simulink model "DDC_decimation"  (R2014b)
settings: Solver=FixedStepDiscrete  SolverMode=SingleTasking  StartTime=0.0  StopTime=4096/fs  RelTol=1e-3
PreLoadFcn:
  | %%%%%%%%%%%%%%%%%%%%%%%%%%%%%%%%%%%%%%%%%%%%%%%%%%%%%%%%%%%%%%%%%%%%%%%%%%%
  | % check to see if Simulink library folder is missing from the MATLAB path %
  | %%%%%%%%%%%%%%%%%%%%%%%%%%%%%%%%%%%%%%%%%%%%%%%%%%%%%%%%%%%%%%%%%%%%%%%%%%%
  | if isempty(strfind(path, 'rtlsdr_book_library'))
  | 
  |     % create error window
  |     fig_error = figure(...
  |         'Name', 'Error: RTL-SDR Book Library',...
  |         'Toolbar','none',...
  |         'MenuBar','none',...
  |         'NumberTitle','off',...
  |         'Resize','off',...
  |         'WindowStyle','modal');
  |     fig_error.Position(3) = 600;
  |     fig_error.Position(4) = 150;
  |     fig_axes = axes(...
  |         'Parent',fig_error,...
  |         'Position',[0,0,1,1],...
  |         'visible','off');
  |     % error message
  |     t_title = text(.05,.8,...
  |         'MISSING DIRECTORIES',...
  |         'FontSize',11.5);
  |     t_body = text(.075,.6,...
  |         [{'Simulink cannot find the  \it{<root>}\rm / \it{rtlsdr\_book\_library}\rm  folder in the \it{MATLAB Path}\rm.'},...
  |         {'Please set the MATLAB path following the instructions given in Exercise 2.4.'}],...
  |         'FontSize',10.5);
  |     % buttons
  |     btn_path = uicontrol(...
  |         'Parent',fig_error,...
  |         'String','Set Path Now',...
  |         'FontSize',10,...
  |         'Callback', 'pathtool; close(fig_error);',...
  |         'Position', [fig_error.Position(3)/2-210, 30, 200, 30]);
  |     btn_abort = uicontrol(...
  |         'Parent',fig_error,...
  |         'String','No thanks',...
  |         'FontSize',10,...
  |         'Callback', 'close(fig_error); abort=1;',...
  |         'Position', [fig_error.Position(3)/2+10, 30, 200, 30]);
  | 
  |     % pause to allow user to interact with error box
  |     uiwait(fig_error);
  | 
  |     % abort simulation
  |     try
  |         if abort==1
  |             set_param(gcs, 'SimulationCommand', 'stop');
  |         end
  |     end
  | 
  |     % if user has set path, allow diagram to be updated
  |     if ~exist('abort','var')
  |         % create error window
  |         fig_update = figure(...
  |             'Name', 'Update Diagram',...
  |             'Toolbar','none',...
  |             'MenuBar','none',...
  |             'NumberTitle','off',...
  |             'Resize','off');
  |         fig_update.Position(3) = 400;
  |         fig_update.Position(4) = 120;
  |         fig_axes = axes(...
  |             'Parent',fig_update,...
  |             'Position',[0,0,1,1],...
  |             'visible','off');
  |         % instruction message
  |         t_body = text(.075,.7,...
  |             'Once you have set the path, update the block diagram',...
  |             'FontSize',10.5);
  |         % button
  |         btn_update = uicontrol(...
  |             'Parent',fig_update,...
  |             'String','Update Block Diagram',...
  |             'FontSize',10,...
  |             'Callback', 'set_param(gcs,''SimulationCommand'',''update''); close(gcf)',...
  |             'Position', [fig_update.Position(3)/2-100, 30, 200, 30]);
  |     end
  | 
  |     % clear error components
  |     clear('fig_error','fig_update','fig_axes','t_title','t_body','btn_path','btn_abort','btn_update','abort');
  | 
  | end
  | %%%%%%%%%%%%%%%%%%%%%%%%%%%%%%%%%%%%%%%%%%%%%%%%%%%%%%%%%%%%%%%%%%%%%%%%%%%
  | 
  | DDC1_setup
  | 
  | % annotations for the pink and purple blocks
  | % going from right to left...
  | 
  | MHz = 100;
  | fs = MHz * 1e6;
  | 
  | fs_CIC_in = fs/CIC_R;
  | MHz_CIC_in = MHz/CIC_R;
  | 
  | fs_CFIR_in = fs/(CIC_R*CFIR_L_factor);
  | MHz_CFIR_in = MHz/(CIC_R*CFIR_L_factor);
  | 
  | fs_RRC_in = fs/(CIC_R*CFIR_L_factor*RRC_L_factor);
  | MHz_RRC_in = MHz/(CIC_R*CFIR_L_factor*RRC_L_factor);
StartFcn:
  | close all;
undefined symbols (not defined in the file): CFIR_L_factor, CIC_R, RRC_L_factor, startfcn_time_scope
libraries: dspmlti4 x12, commdigbbndpm3 x2, dspsigops x2, rtlsdr_book_library x1, dsparch4 x1, commnoisgen2 x1, commrandsrc2 x1
CloseFcn:
  | closefcn_model;
Description:
  | Software, Simulation Examples and Design Exercises Licence Agreement
  | 
  | This license agreement refers to the simulation examples, design exercises and files,
  | and associated software MATLAB and Simulink resources that accompany the book:
  | 
  |      Title: Software Defined Radio using MATLAB & Simulink and the RTL-SDR
  |      Published by Strathclyde Academic Media, 2015
  |      Authored by Robert W. Stewart, Kenneth W. Barlee, Dale S.W. Atkinson,
  |      and Louise H. Crockett
  | 
  | and made available as a download from, www.desktopSDR.com or variously acquired
  | by other means such as via USB storage, cloud storage, disk or any other electronic
  | or optical or magnetic storage mechanism. These files and associated software may
  | be used subject to the terms of agreement of the conditions below:
  | 
  |     Copyright © 2015 Robert W. Stewart, Kenneth W. Barlee, Dale S.W. Atkinson,
  |     and Louise H. Crockett
  |     All rights reserved.
  | 
  | Redistribution and use in source and binary forms, with or without modification, are
  | permitted provided that the following conditions are met:
  | 
  |    1.  Redistributions of source code must retain the above copyright notice, this list of
  |         conditions and the following disclaimer.
  | 
  |    2.  Redistributions in binary form must reproduce the above copyright notice, this
  |         list of conditions and the following disclaimer in the documentation and/or other
  |         materials provided with the distribution.
  | 
  |    3.  Neither the name of the copyright holder nor the names of its contributors may
  |         be used to endorse or promote products derived from this software without
  |         specific prior written permission.
  | 
  |    4.  In all cases, the software is, and all modifications and derivatives of the
  |         software shall be, licensed to you solely for use in conjunction with The
  |         MathWorks, Inc. products and service offerings.
  | 
  | THIS SOFTWARE IS PROVIDED BY THE COPYRIGHT HOLDERS AND CONTRIBUTORS
  | "AS IS" AND ANY EXPRESS OR IMPLIED WARRANTIES, INCLUDING, BUT NOT LIMITED
  | TO, THE IMPLIED WARRANTIES OF MERCHANTABILITY AND FITNESS FOR A
  | PARTICULAR PURPOSE ARE DISCLAIMED. IN NO EVENT SHALL THE COPYRIGHT
  | HOLDER OR CONTRIBUTORS BE LIABLE FOR ANY DIRECT, INDIRECT, INCIDENTAL,
  | SPECIAL, EXEMPLARY, OR CONSEQUENTIAL DAMAGES (INCLUDING, BUT NOT
  | LIMITED TO, PROCUREMENT OF SUBSTITUTE GOODS OR SERVICES; LOSS OF USE,
  | DATA, OR PROFITS; OR BUSINESS INTERRUPTION) HOWEVER CAUSED AND ON ANY
  | THEORY OF LIABILITY, WHETHER IN CONTRACT, STRICT LIABILITY, OR TORT
  | (INCLUDING NEGLIGENCE OR OTHERWISE) ARISING IN ANY WAY OUT OF THE USE
  | OF THIS SOFTWARE, EVEN IF ADVISED OF THE POSSIBILITY OF SUCH DAMAGE.
  | 
  | 
  | Audio Tracks used in Simulations Examples and Design Exercises
  | 
  | The music and vocal files used within the Examples files and software within the book
  | were variously written, arranged, performed, recorded and produced by Garrey Rice,
  | Adam Struth, Jamie Struth, Iain Thistlethwaite and also Marshall Craigmyle who
  | collectively, and individually where appropriate, assert and retain all of their copyright,
  | performance and artistic rights. Permission to use and reproduce this music is
  | granted for all purposes associated with MATLAB and Simulink software and the
  | simulation examples and design exercises files that accompany this book. Requests to
  | use the music for any other purpose should be directed to: info@desktopSDR.com.
  | For information on music track names, full credits, and links to the musicians please
  | refer to www.desktopSDR.com/more/audio.
settings Model: Creator=desktopSDR Team  LastModifiedBy=desktopSDR Team
settings DataIOCC: LimitDataPoints=off  SaveOutput=off  SignalLogging=off  SaveTime=off
settings OptimizationCC: BlockReduction=off  ConditionallyExecuteInputs=off  InlineParams=on
settings DebuggingCC: AlgebraicLoopMsg=error  UnderspecifiedInitializationDetection=Classic  MergeDetectMultiDrivingBlocksExec=none  SingleTaskRateTransMsg=error  ParameterOverflowMsg=warning  StateNameClashWarn=warning
settings HardwareCC: ProdHWDeviceType=ASIC/FPGA->ASIC/FPGA  ProdEqTarget=off

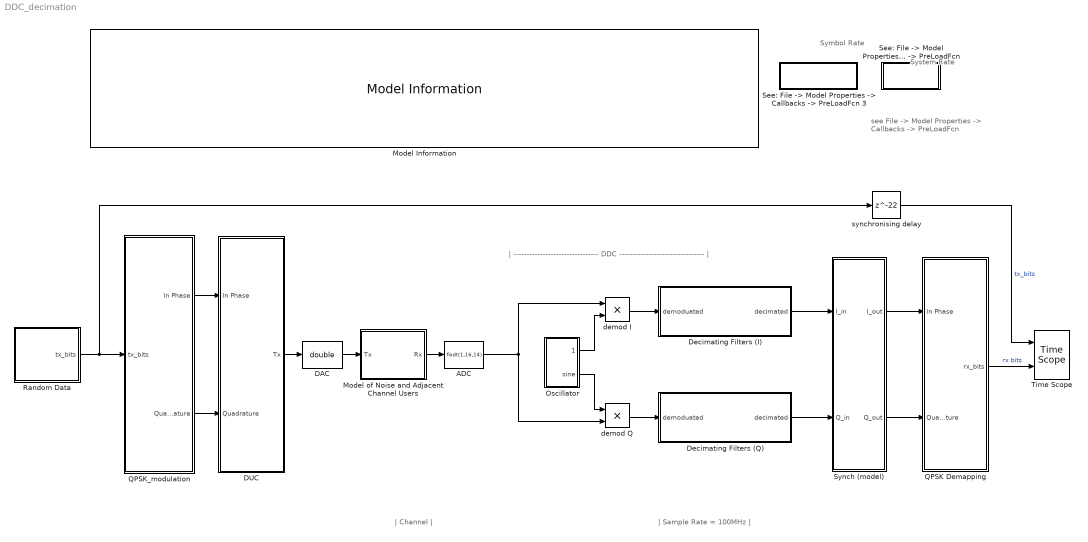
== system DDC_decimation ==
  note: | -------------------------------- DDC -------------------------------- |
  note: System Rate
  note: see File -> Model Properties
      | -> Callbacks -> PreLoadFcn
  note: Symbol Rate
  note: | Sample Rate = 100MHz |
  note: | Channel |
  ADC : DataTypeConversion  OutDataTypeStr=fixdt(1,16,14)
  DAC : DataTypeConversion  OutDataTypeStr=double
  DUC : Subsystem
  Decimating Filters (I) : Subsystem
  Decimating Filters (Q) : Subsystem
  Model Information : rtlsdr_book_library/Additional Tools/Model Information/Model Information
  Model of Noise and Adjacent Channel Users : Subsystem
  Oscillator : Subsystem  mask(Simple Quadrature Oscillator){fc=40e6}
      mask prompts: fc "Frequency"
  QPSK Demapping : Subsystem
  QPSK_modulation : Subsystem
  Random Data : Subsystem
  "See: File -> Model Properties -> Callbacks -> PreLoadFcn " : Subsystem
      mask Display:
      | MHz = evalin('base', 'MHz');
      | fprintf(['fs = ',num2str(MHz),' MHz']);
  "See: File -> Model Properties -> Callbacks -> PreLoadFcn 3" : Subsystem
      mask Display:
      | MHz_RRC_in = evalin('base', 'MHz_RRC_in');
      | fprintf(['fR1 = ',num2str(MHz_RRC_in),' MHz']);
  Synch (model) : Subsystem
  Time Scope : TimeScope  StartFcn=startfcn_time_scope;  DefaultConfigurationName=spbscopes.TimeScopeBlockCfg  NumInputPorts=2
  demod I : Product  OutDataTypeStr=fixdt(1,16,15)
  demod Q : Product  OutDataTypeStr=fixdt(1,16,15)
  synchronising delay : Delay  DelayLength=22  InputProcessing=Columns as channels (frame based)
  wires:
  Random Data/1(tx_bits) -> synchronising delay/1, QPSK_modulation/1(tx_bits)
  ADC/1 -> demod I/1, demod Q/2
  Oscillator/1(cosine) -> demod I/2
  Oscillator/2(sine) -> demod Q/1
  demod I/1 -> Decimating Filters (I)/1(demoduated)
  demod Q/1 -> Decimating Filters (Q)/1(demoduated)
  DAC/1 -> Model of Noise and Adjacent Channel Users/1(Tx)
  QPSK_modulation/1(In Phase) -> DUC/1(In Phase)
  QPSK_modulation/2(Quadrature) -> DUC/2(Quadrature)
  DUC/1(Tx) -> DAC/1
  Model of Noise and Adjacent Channel Users/1(Rx) -> ADC/1
  synchronising delay/1 -> Time Scope/1  "tx_bits"
  QPSK Demapping/1(rx_bits) -> Time Scope/2  "rx bits"
  Decimating Filters (I)/1(" decimated") -> Synch (model)/1(I_in)
  Decimating Filters (Q)/1(" decimated") -> Synch (model)/2(Q_in)
  Synch (model)/1(I_out) -> QPSK Demapping/1(In Phase)
  Synch (model)/2(Q_out) -> QPSK Demapping/2(Quadrature)

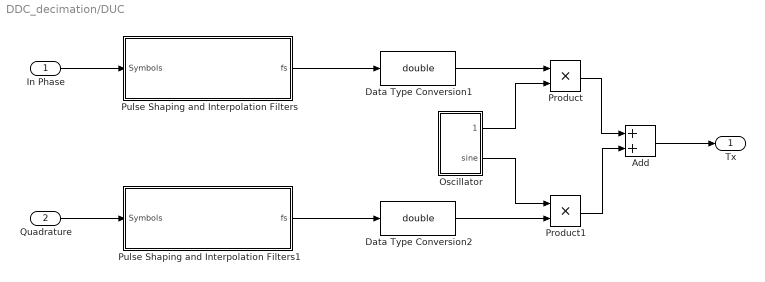
== system DDC_decimation/DUC ==
  In Phase : Inport
  Quadrature : Inport  Port=2
  Add : Sum  OutDataTypeStr=double
  Data Type Conversion1 : DataTypeConversion  OutDataTypeStr=double
  Data Type Conversion2 : DataTypeConversion  OutDataTypeStr=double
  Oscillator : Subsystem  mask(Simple Quadrature Oscillator){fc=40e6}
      mask prompts: fc "Frequency"
  Product : Product  OutDataTypeStr=double
  Product1 : Product  OutDataTypeStr=double
  Pulse Shaping and Interpolation Filters : Subsystem
  Pulse Shaping and Interpolation Filters1 : Subsystem
  Tx : Outport
  wires:
  Add/1 -> Tx/1
  Pulse Shaping and Interpolation Filters/1(" fs") -> Data Type Conversion1/1
  Pulse Shaping and Interpolation Filters1/1(" fs") -> Data Type Conversion2/1
  Oscillator/1(cosine) -> Product/2
  Oscillator/2(sine) -> Product1/1
  Product1/1 -> Add/2
  Product/1 -> Add/1
  Data Type Conversion1/1 -> Product/1
  Data Type Conversion2/1 -> Product1/2
  In Phase/1 -> Pulse Shaping and Interpolation Filters/1(Symbols)
  Quadrature/1 -> Pulse Shaping and Interpolation Filters1/1(Symbols)

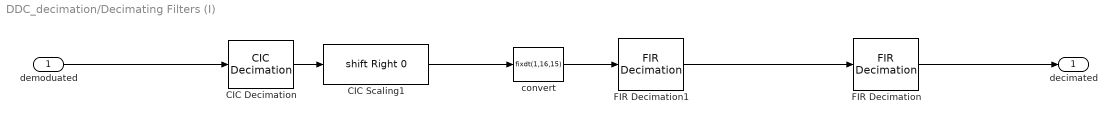
== system DDC_decimation/Decimating Filters (I) ==
  demoduated : Inport
  CIC Decimation : dspmlti4/CIC Decimation  filtFrom=Multirate object in workspace  filtobj=D_hCIC  ftype=Decimator  R=2  M=1  N=2  filterInternals=Full precision  BPS=[16 16 16 16]  FLPS=0  outputWordLength=32  outputFracLength=0  launchFVT=off  framing=Maintain input frame rate  RateOptions=Allow multirate processing
  CIC Scaling1 : ArithShift  BinPtShiftNumber=-10  BitShiftDirection=Right
  FIR Decimation : dspmlti4/FIR Decimation  h=fir1(35,0.4)  D=2  filtStruct=Direct form  framing=Allow multirate processing  inputOffset=0  outputBufInitCond=0  firstCoeffDataTypeStr=Inherit: Same word length as input  firstCoeffLastDataTypeStr=Inherit: Same word length as input  firstCoeffMin=[]  firstCoeffMax=[]  outputDataTypeStr=Inherit: Same as accumulator  outputLastDataTypeStr=Inherit: Same as accumulator  outputMin=[]  outputMax=[]  roundingMode=Floor  overflowMode=off  FilterSource=Filter object  FilterObject=D_hRRC
      settings: allowOverrides=off
  FIR Decimation1 : dspmlti4/FIR Decimation  h=fir1(35,0.4)  D=2  filtStruct=Direct form  framing=Allow multirate processing  inputOffset=0  outputBufInitCond=0  firstCoeffDataTypeStr=Inherit: Same word length as input  firstCoeffLastDataTypeStr=Inherit: Same word length as input  firstCoeffMin=[]  firstCoeffMax=[]  outputDataTypeStr=Inherit: Same as accumulator  outputLastDataTypeStr=Inherit: Same as accumulator  outputMin=[]  outputMax=[]  roundingMode=Floor  overflowMode=off  FilterSource=Filter object  FilterObject=D_hCFIR
      settings: allowOverrides=off
  convert : DataTypeConversion  OutDataTypeStr=fixdt(1,16,15)
  " decimated" : Outport
  wires:
  CIC Decimation/1 -> CIC Scaling1/1
  CIC Scaling1/1 -> convert/1
  FIR Decimation1/1 -> FIR Decimation/1
  demoduated/1 -> CIC Decimation/1
  FIR Decimation/1 -> " decimated"/1
  convert/1 -> FIR Decimation1/1

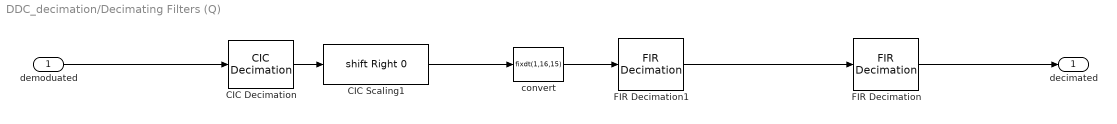
== system DDC_decimation/Decimating Filters (Q) ==
  demoduated : Inport
  CIC Decimation : dspmlti4/CIC Decimation  filtFrom=Multirate object in workspace  filtobj=D_hCIC  ftype=Decimator  R=2  M=1  N=2  filterInternals=Full precision  BPS=[16 16 16 16]  FLPS=0  outputWordLength=32  outputFracLength=0  launchFVT=off  framing=Maintain input frame rate  RateOptions=Allow multirate processing
  CIC Scaling1 : ArithShift  BinPtShiftNumber=-10  BitShiftDirection=Right
  FIR Decimation : dspmlti4/FIR Decimation  h=fir1(35,0.4)  D=2  filtStruct=Direct form  framing=Allow multirate processing  inputOffset=0  outputBufInitCond=0  firstCoeffDataTypeStr=Inherit: Same word length as input  firstCoeffLastDataTypeStr=Inherit: Same word length as input  firstCoeffMin=[]  firstCoeffMax=[]  outputDataTypeStr=Inherit: Same as accumulator  outputLastDataTypeStr=Inherit: Same as accumulator  outputMin=[]  outputMax=[]  roundingMode=Floor  overflowMode=off  FilterSource=Filter object  FilterObject=D_hRRC
      settings: allowOverrides=off
  FIR Decimation1 : dspmlti4/FIR Decimation  h=fir1(35,0.4)  D=2  filtStruct=Direct form  framing=Allow multirate processing  inputOffset=0  outputBufInitCond=0  firstCoeffDataTypeStr=Inherit: Same word length as input  firstCoeffLastDataTypeStr=Inherit: Same word length as input  firstCoeffMin=[]  firstCoeffMax=[]  outputDataTypeStr=Inherit: Same as accumulator  outputLastDataTypeStr=Inherit: Same as accumulator  outputMin=[]  outputMax=[]  roundingMode=Floor  overflowMode=off  FilterSource=Filter object  FilterObject=D_hCFIR
      settings: allowOverrides=off
  convert : DataTypeConversion  OutDataTypeStr=fixdt(1,16,15)
  " decimated" : Outport
  wires:
  FIR Decimation/1 -> " decimated"/1
  demoduated/1 -> CIC Decimation/1
  FIR Decimation1/1 -> FIR Decimation/1
  CIC Scaling1/1 -> convert/1
  CIC Decimation/1 -> CIC Scaling1/1
  convert/1 -> FIR Decimation1/1

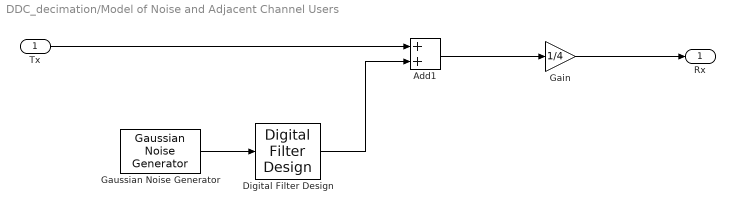
== system DDC_decimation/Model of Noise and Adjacent Channel Users ==
  Tx : Inport
  Add1 : Sum  OutDataTypeStr=fixdt(1,17,14)
  Digital Filter Design : dsparch4/Digital Filter Design  mwdsp_browser_bugfix_var=off
  Gain : Gain  Gain=1/4
  Gaussian Noise Generator : commnoisgen2/Gaussian Noise Generator  m=0  d=1  s=41  Ts=1/fs  frameBased=off  sampPerFrame=1  orient=off  outDataType=double
  Rx : Outport
  wires:
  Tx/1 -> Add1/1
  Gaussian Noise Generator/1 -> Digital Filter Design/1
  Add1/1 -> Gain/1
  Gain/1 -> Rx/1
  Digital Filter Design/1 -> Add1/2

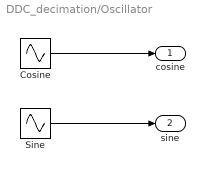
== system DDC_decimation/Oscillator ==
  "Cosine " : Sin  Frequency=fc*2*pi  Phase=pi/2  SampleTime=1/fs
  Sine : Sin  Frequency=fc*2*pi  SampleTime=1/fs
  cosine : Outport
  sine : Outport  Port=2
  wires:
  Sine/1 -> sine/1
  "Cosine "/1 -> cosine/1

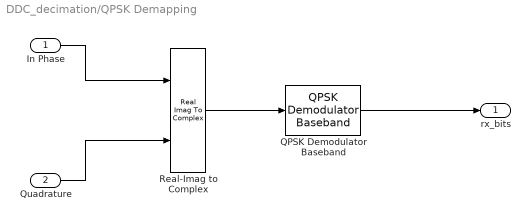
== system DDC_decimation/QPSK Demapping ==
  In Phase : Inport
  Quadrature : Inport  Port=2
  QPSK Demodulator Baseband : commdigbbndpm3/QPSK Demodulator Baseband  Ph=pi/4  Dec=Gray  OutType=Bit  DecType=Hard decision  VarSource=Dialog  Variance=1  outDtype1=Inherit via internal rule  outDtype2=Inherit via internal rule  derotateFactorWordLen=16
  Real-Imag to Complex : RealImagToComplex
  rx_bits : Outport
  wires:
  Quadrature/1 -> Real-Imag to Complex/2
  In Phase/1 -> Real-Imag to Complex/1
  Real-Imag to Complex/1 -> QPSK Demodulator Baseband/1
  QPSK Demodulator Baseband/1 -> rx_bits/1

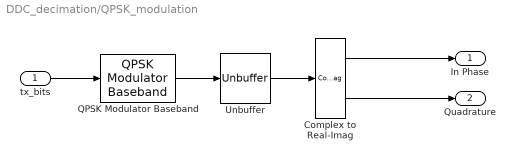
== system DDC_decimation/QPSK_modulation ==
  tx_bits : Inport
  Complex to Real-Imag : ComplexToRealImag
  QPSK Modulator Baseband : commdigbbndpm3/QPSK Modulator Baseband  InType=Bit  Enc=Gray  Ph=pi/4  outDtype=Fixed-point  outWordLen=16  outUDDataType=sfix(16)  outFracLenMode=User-defined  outFracLen=15
  Unbuffer : Unbuffer  SampleBasedProcessing=Same as frame based
  In Phase : Outport
  Quadrature : Outport  Port=2
  wires:
  Complex to Real-Imag/2 -> Quadrature/1
  Complex to Real-Imag/1 -> In Phase/1
  QPSK Modulator Baseband/1 -> Unbuffer/1
  tx_bits/1 -> QPSK Modulator Baseband/1
  Unbuffer/1 -> Complex to Real-Imag/1

== system DDC_decimation/Random Data ==
  Bernoulli Binary Generator : commrandsrc2/Bernoulli Binary Generator  P=0.5  seed=61  Ts=(0.5*CIC_R*RRC_L_factor*CFIR_L_factor)/fs  frameBased=on  sampPerFrame=2  orient=off  outDataType=boolean
  tx_bits : Outport
  wires:
  Bernoulli Binary Generator/1 -> tx_bits/1  "Transmitted Bits"

== system DDC_decimation/See: File -> Model Properties -> Callbacks -> PreLoadFcn  ==

== system DDC_decimation/See: File -> Model Properties -> Callbacks -> PreLoadFcn 3 ==

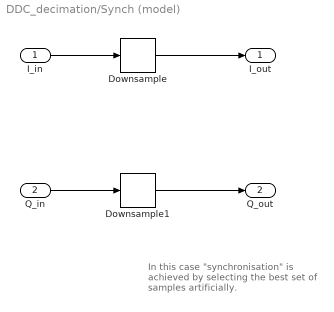
== system DDC_decimation/Synch (model) ==
  note: In this case "synchronisation" is
      | achieved by selecting the best set
      | of samples artificially.
  I_in : Inport
  Q_in : Inport  Port=2
  Downsample : dspsigops/Downsample  N=2  phase=0  RateOptions=Allow multirate processing  smode=Allow multirate  fmode=Maintain input frame size  ic=0
  Downsample1 : dspsigops/Downsample  N=2  phase=0  RateOptions=Allow multirate processing  smode=Allow multirate  fmode=Maintain input frame size  ic=0
  I_out : Outport
  Q_out : Outport  Port=2
  wires:
  I_in/1 -> Downsample/1
  Q_in/1 -> Downsample1/1
  Downsample1/1 -> Q_out/1
  Downsample/1 -> I_out/1

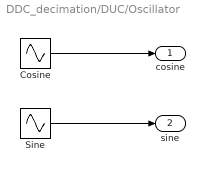
== system DDC_decimation/DUC/Oscillator ==
  "Cosine " : Sin  Frequency=fc*2*pi  Phase=pi/2  SampleTime=1/fs
  Sine : Sin  Frequency=fc*2*pi  SampleTime=1/fs
  cosine : Outport
  sine : Outport  Port=2
  wires:
  Sine/1 -> sine/1
  "Cosine "/1 -> cosine/1

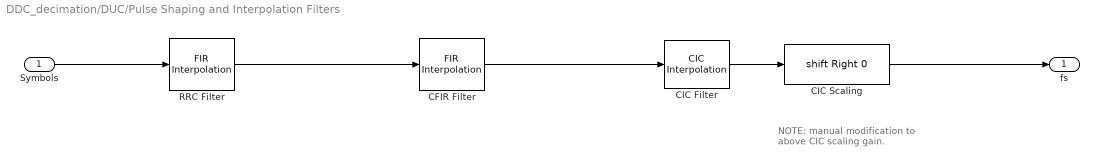
== system DDC_decimation/DUC/Pulse Shaping and Interpolation Filters ==
  note: NOTE: manual modification
      |  to above CIC scaling gain.
  Symbols : Inport
  CFIR Filter : dspmlti4/FIR Interpolation  h=fir1(15,1/4)  L=3  framing=Allow multirate processing  outputBufInitCond=0  firstCoeffDataTypeStr=Inherit: Same word length as input  firstCoeffLastDataTypeStr=Inherit: Same word length as input  firstCoeffMin=[]  firstCoeffMax=[]  outputDataTypeStr=Inherit: Same as accumulator  outputLastDataTypeStr=Inherit: Same as accumulator  outputMin=[]  outputMax=[]  roundingMode=Floor  overflowMode=off  FilterSource=Filter object  FilterObject=hCFIR
  CIC Filter : dspmlti4/CIC Interpolation  filtFrom=Multirate object in workspace  filtobj=hCIC  ftype=Interpolator  R=2  M=1  N=2  filterInternals=Full precision  BPS=[16 16 16 16]  FLPS=0  outputWordLength=32  outputFracLength=0  launchFVT=off  framing=Allow multirate processing
  CIC Scaling : ArithShift  BinPtShiftNumber=-12  BitShiftDirection=Right
  RRC Filter : dspmlti4/FIR Interpolation  h=fir1(15,1/4)  L=3  framing=Allow multirate processing  outputBufInitCond=0  firstCoeffDataTypeStr=Inherit: Same word length as input  firstCoeffLastDataTypeStr=Inherit: Same word length as input  firstCoeffMin=[]  firstCoeffMax=[]  outputDataTypeStr=Inherit: Same as accumulator  outputLastDataTypeStr=Inherit: Same as accumulator  outputMin=[]  outputMax=[]  roundingMode=Floor  overflowMode=off  FilterSource=Filter object  FilterObject=hRRC
  " fs" : Outport
  wires:
  RRC Filter/1 -> CFIR Filter/1
  Symbols/1 -> RRC Filter/1
  CIC Filter/1 -> CIC Scaling/1
  CIC Scaling/1 -> " fs"/1
  CFIR Filter/1 -> CIC Filter/1

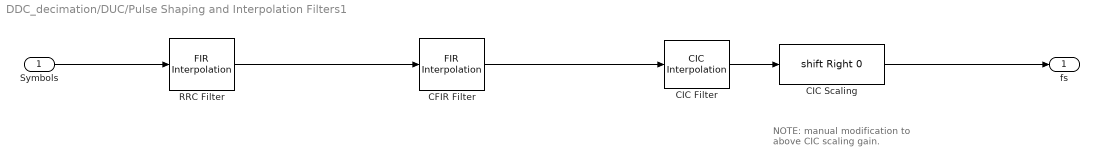
== system DDC_decimation/DUC/Pulse Shaping and Interpolation Filters1 ==
  note: NOTE: manual modification
      |  to above CIC scaling gain.
  Symbols : Inport
  CFIR Filter : dspmlti4/FIR Interpolation  h=fir1(15,1/4)  L=3  framing=Allow multirate processing  outputBufInitCond=0  firstCoeffDataTypeStr=Inherit: Same word length as input  firstCoeffLastDataTypeStr=Inherit: Same word length as input  firstCoeffMin=[]  firstCoeffMax=[]  outputDataTypeStr=Inherit: Same as accumulator  outputLastDataTypeStr=Inherit: Same as accumulator  outputMin=[]  outputMax=[]  roundingMode=Floor  overflowMode=off  FilterSource=Filter object  FilterObject=hCFIR
  CIC Filter : dspmlti4/CIC Interpolation  filtFrom=Multirate object in workspace  filtobj=hCIC  ftype=Interpolator  R=2  M=1  N=2  filterInternals=Full precision  BPS=[16 16 16 16]  FLPS=0  outputWordLength=32  outputFracLength=0  launchFVT=off  framing=Allow multirate processing
  CIC Scaling : ArithShift  BinPtShiftNumber=-12  BitShiftDirection=Right
  RRC Filter : dspmlti4/FIR Interpolation  h=fir1(15,1/4)  L=3  framing=Allow multirate processing  outputBufInitCond=0  firstCoeffDataTypeStr=Inherit: Same word length as input  firstCoeffLastDataTypeStr=Inherit: Same word length as input  firstCoeffMin=[]  firstCoeffMax=[]  outputDataTypeStr=Inherit: Same as accumulator  outputLastDataTypeStr=Inherit: Same as accumulator  outputMin=[]  outputMax=[]  roundingMode=Floor  overflowMode=off  FilterSource=Filter object  FilterObject=hRRC
  " fs" : Outport
  wires:
  CFIR Filter/1 -> CIC Filter/1
  CIC Scaling/1 -> " fs"/1
  CIC Filter/1 -> CIC Scaling/1
  Symbols/1 -> RRC Filter/1
  RRC Filter/1 -> CFIR Filter/1
